simulink model "ModelAndSystem"  (R2017b)
settings: Solver=ode8  StartTime=0.0  StopTime=5  FixedStep=0.01  RelTol=1e-3
undefined symbols (not defined in the file or in its folder): V
settings Model: Creator=labadmin  LastModifiedBy=labadmin
settings RTWCC: SystemTargetFile=sldrt.tlc  TemplateMakefile=sldrt.tmf  Description=Simulink Desktop Real-Time  RTWCompilerOptimization=on
settings CodeAppCC: MaxIdLength=95
settings SimulinkDesktopRealTimeCC: TargetPreCompLibLocation=C:\Program Files\MATLAB\R2017b\toolbox\sldrt\lib\win64

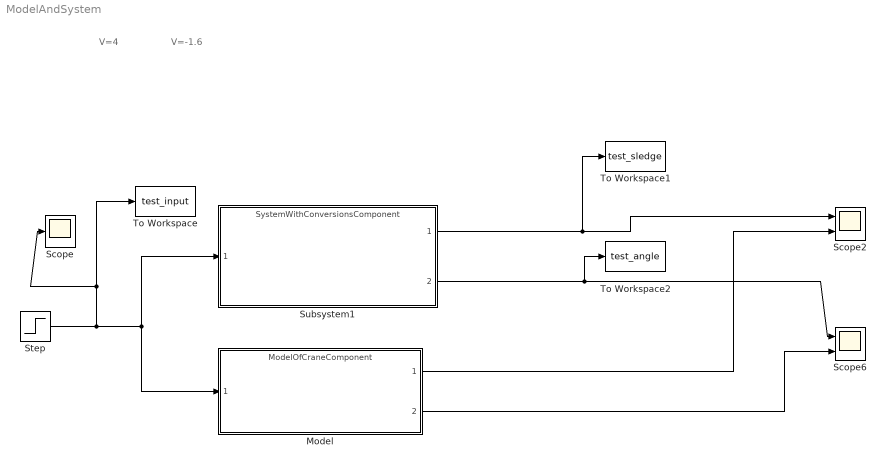
== system ModelAndSystem ==
  note: V=4
  note: V=-1.6
  Model : ModelReference  ModelNameDialog=ModelOfCraneComponent.slx  SimulationMode=Normal  ModelReferenceVersion=1.7
  Scope : Scope
  Scope2 : Scope  NumInputPorts=2
  Scope6 : Scope  NumInputPorts=2
  Step : Step  Time=0  After=V  SampleTime=0
  Subsystem1 : ModelReference  ModelNameDialog=SystemWithConversionsComponent  SimulationMode=Normal  ModelReferenceVersion=1.13
  To Workspace : ToWorkspace  VariableName=test_input  SaveFormat=Timeseries  SampleTime=-1
  To Workspace1 : ToWorkspace  VariableName=test_sledge  SaveFormat=Timeseries  SampleTime=-1
  To Workspace2 : ToWorkspace  VariableName=test_angle  SaveFormat=Timeseries  SampleTime=-1
  wires:
  Step/1 -> Scope/1, To Workspace/1, Model/1, Subsystem1/1
  Model/1 -> Scope2/2
  Model/2 -> Scope6/2
  Subsystem1/1 -> To Workspace1/1, Scope2/1
  Subsystem1/2 -> To Workspace2/1, Scope6/1
